simulink model "sv1_0"  (R2022b)
settings: Solver=VariableStepAuto  StartTime=0.0  StopTime=10.0  RelTol=1e-3
values from neighbouring files (symbols this model uses):
  m = rotation_matrix([0 0 1], theta)    [ectopic.m]    (also in ectopic_dirty_1.m; workspace.m)
undefined symbols (not defined in the file or in its folder): X, Y, Z
libraries: sm_lib x67, nesl_utility x1
(part 1 of 2)
settings Model: Creator=谢兴彪  LastModifiedBy=谢兴彪

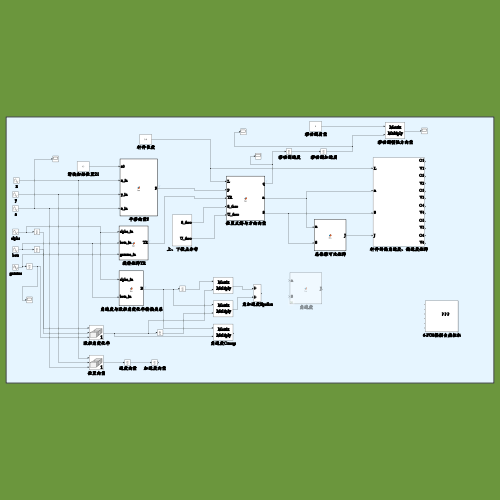
[thumbnail: Simulink's stored preview of the top-level diagram]
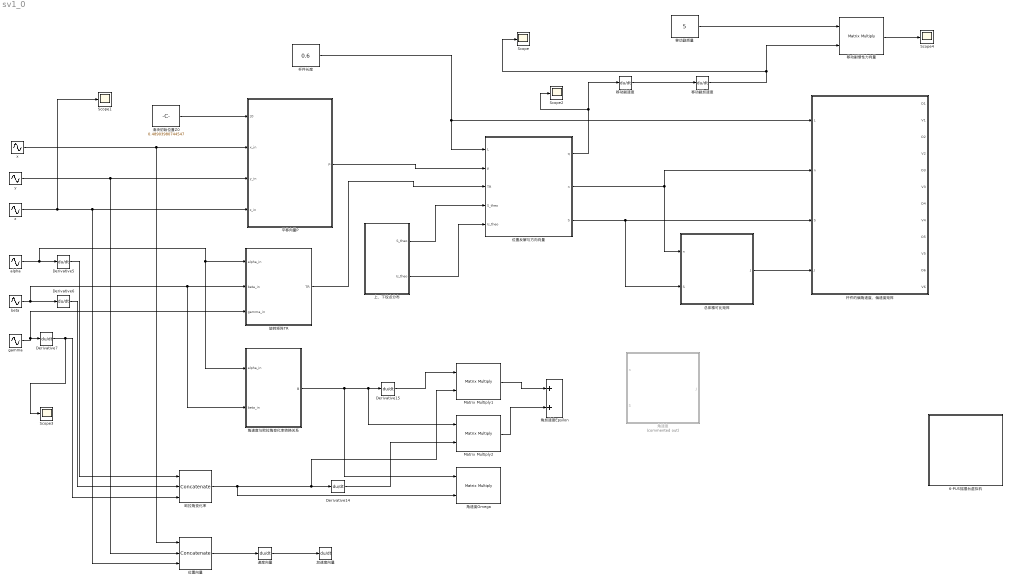
== system sv1_0 ==
  6-PUS摇摆台虚拟机 : Subsystem
      mask Display: image('C:\Users\谢兴彪\Desktop\微信图片_20230811154149.png'); % 使用工具条上的 "编辑图像" 进行更改。
  Derivative{5..7,14..15} (5 alike) : Derivative
  Matrix Multiply1 : Product  Inputs=**  Multiplication=Matrix(*)
  Matrix Multiply2 : Product  Inputs=**  Multiplication=Matrix(*)
  Scope{,1..4} (5 alike) : Scope
  alpha : Sin  Amplitude=0  Frequency=2*pi  SampleTime=0
  beta : Sin  Amplitude=0  Frequency=2*pi  SampleTime=0
  gamma : Sin  Amplitude=0.1  Frequency=2*pi  SampleTime=0.01
  x : Sin  Amplitude=0  Frequency=2*pi  SampleTime=0
  y : Sin  Amplitude=0  Frequency=2*pi  SampleTime=0
  z : Sin  Amplitude=0  Frequency=2  SampleTime=0
  上、下铰点分布 : Subsystem
  位置反解与方向向量 : MATLAB Function  TreatAsAtomicUnit=on
  位置向量 : Concatenate  NumInputs=3  Mode=Multidimensional array
  加速度向量 : Derivative
  平移向量P : MATLAB Function  TreatAsAtomicUnit=on
  总体雅可比矩阵 : MATLAB Function  TreatAsAtomicUnit=on
  旋转矩阵TR : MATLAB Function  TreatAsAtomicUnit=on
  杆件的偏角速度、偏速度矩阵 : Subsystem
  杆件长度 : Constant  Value=0.6
  欧拉角变化率 : Concatenate  NumInputs=3  Mode=Multidimensional array
  滑块初始位置Z0 : Constant  Value=0.48903980744547
  移动副加速度 : Derivative
  移动副惯性力向量 : Product  Inputs=**  Multiplication=Matrix(*)
  移动副质量 : Constant  Value=5
  移动副速度 : Derivative
  角加速度Epsilon : Sum
  角速度 : MATLAB Function  Commented=on  TreatAsAtomicUnit=on
  角速度Omega : Product  Inputs=**  Multiplication=Matrix(*)
  角速度与欧拉角变化率转换关系 : MATLAB Function  TreatAsAtomicUnit=on
  速度向量 : Derivative
  wires:
  滑块初始位置Z0/1 -> 平移向量P/1(z0)
  平移向量P/1(p) -> 位置反解与方向向量/2(p)
  旋转矩阵TR/1(TR) -> 位置反解与方向向量/3(TR)
  上、下铰点分布/1(S_theo) -> 位置反解与方向向量/4(S_theo)
  上、下铰点分布/2(U_theo) -> 位置反解与方向向量/5(U_theo)
  杆件长度/1 -> 位置反解与方向向量/1(L), 杆件的偏角速度、偏速度矩阵/1(L)
  位置反解与方向向量/1(q) -> 移动副速度/1, Scope2/1
  移动副速度/1 -> 移动副加速度/1
  z/1 -> Scope1/1, 位置向量/3, 平移向量P/4(z_in)
  y/1 -> 位置向量/2, 平移向量P/3(y_in)
  x/1 -> 平移向量P/2(x_in), 位置向量/1
  alpha/1 -> 角速度与欧拉角变化率转换关系/1(alpha_in), 旋转矩阵TR/1(alpha_in), Derivative5/1
  beta/1 -> 角速度与欧拉角变化率转换关系/2(beta_in), 旋转矩阵TR/2(beta_in), Derivative6/1
  gamma/1 -> 旋转矩阵TR/3(gamma_in), Derivative7/1
  Derivative5/1 -> 欧拉角变化率/1
  Derivative6/1 -> 欧拉角变化率/2
  Derivative7/1 -> Scope3/1, 欧拉角变化率/3
  欧拉角变化率/1 -> 角速度Omega/2, Matrix Multiply1/2, Derivative14/1
  Derivative14/1 -> Matrix Multiply2/2
  角速度与欧拉角变化率转换关系/1(B) -> Matrix Multiply2/1, Derivative15/1, 角速度Omega/1
  Derivative15/1 -> Matrix Multiply1/1
  Matrix Multiply1/1 -> 角加速度Epsilon/1
  Matrix Multiply2/1 -> 角加速度Epsilon/2
  位置向量/1 -> 速度向量/1
  速度向量/1 -> 加速度向量/1
  位置反解与方向向量/3(S) -> 总体雅可比矩阵/2(S), 杆件的偏角速度、偏速度矩阵/3(S)
  位置反解与方向向量/2(n) -> 杆件的偏角速度、偏速度矩阵/2(n), 总体雅可比矩阵/1(n)
  移动副质量/1 -> 移动副惯性力向量/1
  移动副加速度/1 -> 移动副惯性力向量/2, Scope/1
  总体雅可比矩阵/1(J) -> 杆件的偏角速度、偏速度矩阵/4(J)
  移动副惯性力向量/1 -> Scope4/1

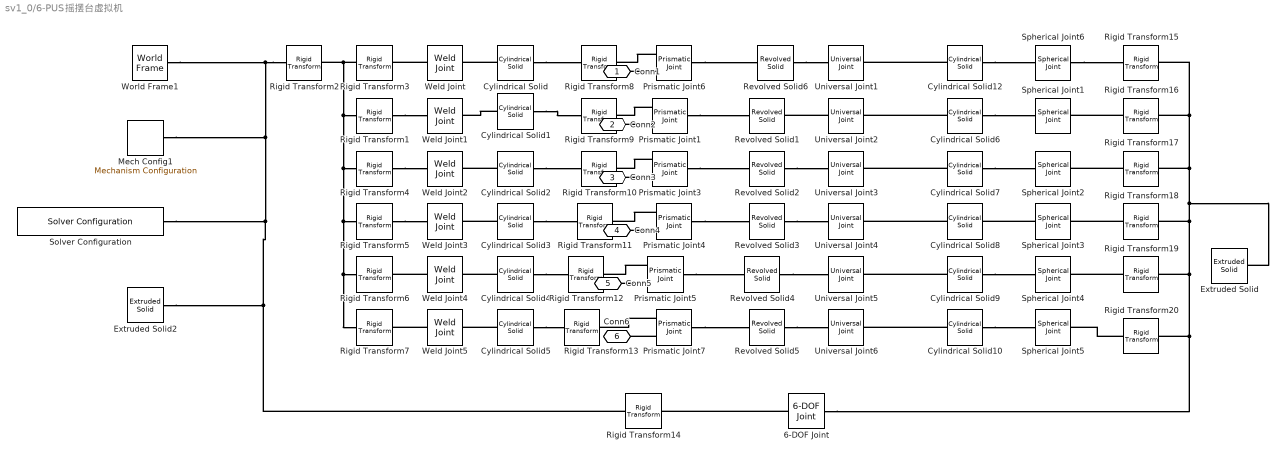
== system sv1_0/6-PUS摇摆台虚拟机 ==
  6-DOF Joint : sm_lib/Joints/6-DOF Joint  JointMode=Normal  SenseConstraintForce=off  SenseConstraintForceX=off  SenseConstraintForceY=off  SenseConstraintForceZ=off  SenseConstraintTorque=off  SenseConstraintTorqueX=off  SenseConstraintTorqueY=off  SenseConstraintTorqueZ=off  SenseTotalForce=off  SenseTotalForceX=off  SenseTotalForceY=off  SenseTotalForceZ=off  SenseTotalTorque=off  SenseTotalTorqueX=off  SenseTotalTorqueY=off  SenseTotalTorqueZ=off  CompositeWrenchDir=FollowerOnBase  CompositeWrenchFrame=BaseFrame  PxEquilibriumPosition=0  PxEquilibriumPositionUnits=m  PxSpringStiffness=0  PxSpringStiffnessUnits=N/m  PxDampingCoefficient=0  PxDampingCoefficientUnits=N/(m/s)  PxTorqueActuationMode=NoTorque  PxMotionActuationMode=ComputedMotion  PxSensePosition=off  PxSenseVelocity=off  PxSenseAcceleration=off  PxSenseTorqueForce=off  PxSenseLowerLimitTorqueForce=off  PxSenseUpperLimitTorqueForce=off  PxLowerLimitSpecify=off  PxLowerLimitBound=-1  PxLowerLimitBoundUnits=m  PxLowerLimitStiffness=1e6  PxLowerLimitStiffnessUnits=N/m  PxLowerLimitDamping=1e3  PxLowerLimitDampingUnits=N/(m/s)  PxLowerLimitTransitionRegionWidth=1e-4  PxLowerLimitTransitionRegionWidthUnits=m  PxUpperLimitSpecify=off  PxUpperLimitBound=1  PxUpperLimitBoundUnits=m  PxUpperLimitStiffness=1e6  PxUpperLimitStiffnessUnits=N/m  PxUpperLimitDamping=1e3  PxUpperLimitDampingUnits=N/(m/s)  PxUpperLimitTransitionRegionWidth=1e-4  PxUpperLimitTransitionRegionWidthUnits=m  PxPositionTargetSpecify=off  PxPositionTargetPriority=High  PxPositionTargetValue=0  PxPositionTargetValueUnits=m  PxVelocityTargetSpecify=off  PxVelocityTargetPriority=High  PxVelocityTargetValue=0  PxVelocityTargetValueUnits=m/s  PyEquilibriumPosition=0  PyEquilibriumPositionUnits=m  PySpringStiffness=0  PySpringStiffnessUnits=N/m  PyDampingCoefficient=0  PyDampingCoefficientUnits=N/(m/s)  PyTorqueActuationMode=NoTorque  PyMotionActuationMode=ComputedMotion  PySensePosition=off  PySenseVelocity=off  PySenseAcceleration=off  PySenseTorqueForce=off  PySenseLowerLimitTorqueForce=off  PySenseUpperLimitTorqueForce=off  PyLowerLimitSpecify=off  PyLowerLimitBound=-1  PyLowerLimitBoundUnits=m  PyLowerLimitStiffness=1e6  PyLowerLimitStiffnessUnits=N/m  PyLowerLimitDamping=1e3  PyLowerLimitDampingUnits=N/(m/s)  PyLowerLimitTransitionRegionWidth=1e-4  PyLowerLimitTransitionRegionWidthUnits=m  PyUpperLimitSpecify=off  PyUpperLimitBound=1  PyUpperLimitBoundUnits=m  PyUpperLimitStiffness=1e6  PyUpperLimitStiffnessUnits=N/m  PyUpperLimitDamping=1e3  PyUpperLimitDampingUnits=N/(m/s)  PyUpperLimitTransitionRegionWidth=1e-4  PyUpperLimitTransitionRegionWidthUnits=m  PyPositionTargetSpecify=off  PyPositionTargetPriority=High  PyPositionTargetValue=0  PyPositionTargetValueUnits=m  PyVelocityTargetSpecify=off  PyVelocityTargetPriority=High  PyVelocityTargetValue=0  PyVelocityTargetValueUnits=m/s  PzEquilibriumPosition=0  PzEquilibriumPositionUnits=m  PzSpringStiffness=0  PzSpringStiffnessUnits=N/m  PzDampingCoefficient=0  PzDampingCoefficientUnits=N/(m/s)  PzTorqueActuationMode=NoTorque  PzMotionActuationMode=ComputedMotion  PzSensePosition=off  PzSenseVelocity=off  PzSenseAcceleration=off  PzSenseTorqueForce=off  PzSenseLowerLimitTorqueForce=off  PzSenseUpperLimitTorqueForce=off  PzLowerLimitSpecify=off  PzLowerLimitBound=-1  PzLowerLimitBoundUnits=m  PzLowerLimitStiffness=1e6  PzLowerLimitStiffnessUnits=N/m  PzLowerLimitDamping=1e3  PzLowerLimitDampingUnits=N/(m/s)  PzLowerLimitTransitionRegionWidth=1e-4  PzLowerLimitTransitionRegionWidthUnits=m  PzUpperLimitSpecify=off  PzUpperLimitBound=1  PzUpperLimitBoundUnits=m  PzUpperLimitStiffness=1e6  PzUpperLimitStiffnessUnits=N/m  PzUpperLimitDamping=1e3  PzUpperLimitDampingUnits=N/(m/s)  PzUpperLimitTransitionRegionWidth=1e-4  PzUpperLimitTransitionRegionWidthUnits=m  PzPositionTargetSpecify=off  PzPositionTargetPriority=High  PzPositionTargetValue=0  PzPositionTargetValueUnits=m  PzVelocityTargetSpecify=off  PzVelocityTargetPriority=High  PzVelocityTargetValue=0  PzVelocityTargetValueUnits=m/s  SphEqPosRotationMethod=None  SphEqPosRotationAngleUnits=deg  SphEqPosRotationStandardAxis=+Z  SphEqPosRotationAngle=0.0  SphEqPosRotationArbitraryAxis=[0 0 1]  SphEqPosFollAlignAxisA=+X  SphEqPosBaseAlignAxisA=+Y  SphEqPosFollAlignAxisB=+Y  SphEqPosBaseAlignAxisB=+Z  SphEqPosRotationSequenceAxes=FollowerAxes  SphEqPosRotationSequence=XYX  SphEqPosRotationSequenceAngles=[0 0 0]  SphEqPosRotationSequenceAnglesUnits=deg  SphEqPosRotationMatrix=[1 0 0; 0 1 0; 0 0 1]  SphEqPosQuaternion=[1 0 0 0]  SphSpringStiffness=0  SphSpringStiffnessUnits=N*m/deg  SphDampingCoefficient=0  SphDampingCoefficientUnits=N*m/(deg/s)  SphActuateTorqueX=off  SphActuateTorqueY=off  SphActuateTorqueZ=off  SphActuateTorque=off  SphTorqueActuationMode=NoTorque  SphMotionActuationMode=ComputedMotion  SphActuationFrame=BaseFrame  SphSensePosition=off  SphSenseVelocityX=off  SphSenseVelocityY=off  SphSenseVelocityZ=off  SphSenseVelocity=off  SphSenseAccelerationX=off  SphSenseAccelerationY=off  SphSenseAccelerationZ=off  SphSenseAcceleration=off  SphSenseTorqueX=off  SphSenseTorqueY=off  SphSenseTorqueZ=off  SphSenseTorqueForce=off  SphSenseLowerLimitTorqueMag=off  SphSenseUpperLimitTorqueMag=off  SphSensingFrame=BaseFrame  SphLowerLimitSpecify=off  SphLowerLimitBound=15  SphLowerLimitBoundUnits=deg  SphLowerLimitStiffness=1e4  SphLowerLimitStiffnessUnits=N*m/deg  SphLowerLimitDamping=10  SphLowerLimitDampingUnits=N*m/(deg/s)  SphLowerLimitTransitionRegionWidth=0.1  SphLowerLimitTransitionRegionWidthUnits=deg  SphUpperLimitSpecify=off  SphUpperLimitBound=45  SphUpperLimitBoundUnits=deg  SphUpperLimitStiffness=1e4  SphUpperLimitStiffnessUnits=N*m/deg  SphUpperLimitDamping=10  SphUpperLimitDampingUnits=N*m/(deg/s)  SphUpperLimitTransitionRegionWidth=0.1  SphUpperLimitTransitionRegionWidthUnits=deg  SphPositionTargetRotationMethod=None  SphPositionTargetRotationAngleUnits=deg  SphPositionTargetRotationStandardAxis=+Z  SphPositionTargetRotationAngle=0.0  SphPositionTargetRotationArbitraryAxis=[0 0 1]  SphPositionTargetFollAlignAxisA=+X  SphPositionTargetBaseAlignAxisA=+Y  SphPositionTargetFollAlignAxisB=+Y  SphPositionTargetBaseAlignAxisB=+Z  SphPositionTargetRotationSequenceAxes=FollowerAxes  SphPositionTargetRotationSequence=XYX  SphPositionTargetRotationSequenceAngles=[0 0 0]  SphPositionTargetRotationSequenceAnglesUnits=deg  SphPositionTargetRotationMatrix=[1 0 0; 0 1 0; 0 0 1]  SphPositionTargetQuaternion=[1 0 0 0]  SphPositionTargetSpecify=off  SphPositionTargetPriority=High  SphVelocityTargetValue=[0 0 0]  SphVelocityTargetValueUnits=deg/s  SphVelocityTargetSpecify=off  SphVelocityTargetPriority=High  SphVelocityTargetInFollowerFrame=on
  Cylindrical Solid{,1..5} (6 alike) : sm_lib/Body Elements/Cylindrical Solid  GraphicAmbientColor=[0.15 0.15 0.15 1.0]  BasedOnType=Density  CenterOfMass=[0 0 0]  CenterOfMassUnits=m  GraphicDiffuseColor=[1 0.4 0.0]  CylinderLength=536.5  CylinderLengthUnits=mm  CylinderRadius=7.5  CylinderRadiusUnits=mm  Density=1000  DensityUnits=kg/m^3  DoExposeReferenceFrame=off  GraphicEmissiveColor=[0.0 0.0 0.0 1.0]  ExportEntireGeometry=off  SerializedFrames=<Frames><Frame><Id>Frame1</Id><Value><Name>F1</Name><Origin><Source>GeometricFeature</Source><FeatureName>bottom curve</FeatureName></Origin><PrimaryAxis><DefinedDirection>+Z</DefinedDirection><Source>ReferenceFrame</Source><SourceDirection>+Z</SourceDirection><FeatureName></FeatureName></PrimaryAxis><SecondaryAxis><DefinedDirection>+X</DefinedDirection><Source>ReferenceFrame</Source><SourceDirection>+X</SourceDirection><FeatureName></FeatureName></SecondaryAxis></Value></Frame><Frame><Id>Frame2</Id><Value><Name>F2</Name><Origin><Source>GeometricFeature</Source><FeatureName>top surface</FeatureName></Origin><PrimaryAxis><DefinedDirection>+Z</DefinedDirection><Source>ReferenceFrame</Source><SourceDirection>+Z</SourceDirection><FeatureName></FeatureName></PrimaryAxis><SecondaryAxis><DefinedDirection>+X</DefinedDirection><Source>ReferenceFrame</Source><SourceDirection>+X</SourceDirection><FeatureName></FeatureName></SecondaryAxis></Value></Frame></Frames>  MarkerShape=Sphere  MarkerSize=10  GraphicType=FromGeometry  InertiaType=CalculateFromGeometry  Mass=1  MassUnits=kg  MomentsOfInertia=[1 1 1]  MomentsOfInertiaUnits=kg*m^2  GraphicOpacity=1.0  ProductsOfInertia=[0 0 0]  ProductsOfInertiaUnits=kg*m^2  GraphicShininess=75  GraphicSpecularColor=[0.5 0.5 0.5 1.0]  GraphicVisPropType=SimpleVisualProperties
  Cylindrical Solid{6..10,12} (6 alike) : sm_lib/Body Elements/Cylindrical Solid  GraphicAmbientColor=[0.15 0.15 0.15 1.0]  BasedOnType=Density  CenterOfMass=[0 0 0]  CenterOfMassUnits=m  GraphicDiffuseColor=[1.0 0.2 0.0]  CylinderLength=600  CylinderLengthUnits=mm  CylinderRadius=20  CylinderRadiusUnits=mm  Density=1000  DensityUnits=kg/m^3  DoExposeReferenceFrame=off  GraphicEmissiveColor=[0.0 0.0 0.0 1.0]  ExportEntireGeometry=off  SerializedFrames=<Frames><Frame><Id>Frame1</Id><Value><Name>F1</Name><Origin><Source>GeometricFeature</Source><FeatureName>bottom curve</FeatureName></Origin><PrimaryAxis><DefinedDirection>+Z</DefinedDirection><Source>ReferenceFrame</Source><SourceDirection>+Z</SourceDirection><FeatureName></FeatureName></PrimaryAxis><SecondaryAxis><DefinedDirection>+X</DefinedDirection><Source>ReferenceFrame</Source><SourceDirection>+X</SourceDirection><FeatureName></FeatureName></SecondaryAxis></Value></Frame><Frame><Id>Frame2</Id><Value><Name>F2</Name><Origin><Source>GeometricFeature</Source><FeatureName>top surface</FeatureName></Origin><PrimaryAxis><DefinedDirection>+Z</DefinedDirection><Source>ReferenceFrame</Source><SourceDirection>+Z</SourceDirection><FeatureName></FeatureName></PrimaryAxis><SecondaryAxis><DefinedDirection>+X</DefinedDirection><Source>ReferenceFrame</Source><SourceDirection>+X</SourceDirection><FeatureName></FeatureName></SecondaryAxis></Value></Frame></Frames>  MarkerShape=Sphere  MarkerSize=10  GraphicType=FromGeometry  InertiaType=CalculateFromGeometry  Mass=1  MassUnits=kg  MomentsOfInertia=[1 1 1]  MomentsOfInertiaUnits=kg*m^2  GraphicOpacity=1.0  ProductsOfInertia=[0 0 0]  ProductsOfInertiaUnits=kg*m^2  GraphicShininess=75  GraphicSpecularColor=[0.5 0.5 0.5 1.0]  GraphicVisPropType=SimpleVisualProperties
  Extruded Solid : sm_lib/Body Elements/Extruded Solid  GraphicAmbientColor=[0.15 0.15 0.15 1.0]  BasedOnType=Density  CenterOfMass=[0 0 0]  CenterOfMassUnits=m  GraphicDiffuseColor=[0 0.1 1]  ExportConvexHullGeometry=off  ExtrusionCrossSection=|  ExtrusionCrossSectionUnits=m  Density=1000  DensityUnits=kg/m^3  DoExposeReferenceFrame=on  GraphicEmissiveColor=[0.0 0.0 0.0 0.3]  ExportEntireGeometry=off  ExtrusionLength=0.025  ExtrusionLengthUnits=m  ExtrusionType=General  SerializedFrames=<Frames/>  MarkerShape=Sphere  MarkerSize=10  GraphicType=FromGeometry  InertiaType=CalculateFromGeometry  Mass=1  MassUnits=kg  MomentsOfInertia=[1 1 1]  MomentsOfInertiaUnits=kg*m^2  PolygonNumSides=6  GraphicOpacity=1.0  PolygonOuterRadius=0.16  PolygonOuterRadiusUnits=m  ProductsOfInertia=[0 0 0]  ProductsOfInertiaUnits=kg*m^2  GraphicShininess=75  GraphicSpecularColor=[0.5 0.5 0.5 1.0]  GraphicVisPropType=AdvancedVisualProperties
      | [0.1373 0.1314; 
      | -0.1373 0.1314; 
      | -0.1824 0.0532; 
      | -0.0451 -0.1846;
      | 0.0451 -0.1846;
      | 0.1824 0.0532]
  Extruded Solid2 : sm_lib/Body Elements/Extruded Solid  GraphicAmbientColor=[0.15 0.15 0.15 1.0]  BasedOnType=Density  CenterOfMass=[0 0 0]  CenterOfMassUnits=m  GraphicDiffuseColor=[1 0.4 0]  ExportConvexHullGeometry=off  ExtrusionCrossSection=|  ExtrusionCrossSectionUnits=m  Density=1000  DensityUnits=kg/m^3  DoExposeReferenceFrame=on  GraphicEmissiveColor=[0.0 0.0 0.0 0.3]  ExportEntireGeometry=off  ExtrusionLength=0.2  ExtrusionLengthUnits=m  ExtrusionType=General  SerializedFrames=<Frames/>  MarkerShape=Sphere  MarkerSize=10  GraphicType=FromGeometry  InertiaType=CalculateFromGeometry  Mass=1  MassUnits=kg  MomentsOfInertia=[1 1 1]  MomentsOfInertiaUnits=kg*m^2  PolygonNumSides=6  GraphicOpacity=1.0  PolygonOuterRadius=0.16  PolygonOuterRadiusUnits=m  ProductsOfInertia=[0 0 0]  ProductsOfInertiaUnits=kg*m^2  GraphicShininess=75  GraphicSpecularColor=[0.5 0.5 0.5 1.0]  GraphicVisPropType=AdvancedVisualProperties
      | [0.1096 0.4878; 
      | -0.1096 0.4878; 
      | -0.4773 -0.1490; 
      | -0.3677 -0.3388;
      | 0.3677 -0.3388;
      | 0.4773 -0.1490]
  Mech Config1 : sm_lib/Utilities/Mechanism Configuration  UniformGravity=None  GravityVector=[0 0 -9.80665]  GravityUnits=m/s^2  LinearizationDelta=0.001  JointModeTransitionNonlinearIterations=2
  Prismatic Joint{1,3..7} (6 alike) : sm_lib/Joints/Prismatic Joint  JointMode=Normal  SenseConstraintForce=off  SenseConstraintForceX=off  SenseConstraintForceY=off  SenseConstraintForceZ=off  SenseConstraintTorque=off  SenseConstraintTorqueX=off  SenseConstraintTorqueY=off  SenseConstraintTorqueZ=off  SenseTotalForce=off  SenseTotalForceX=off  SenseTotalForceY=off  SenseTotalForceZ=off  SenseTotalTorque=off  SenseTotalTorqueX=off  SenseTotalTorqueY=off  SenseTotalTorqueZ=off  CompositeWrenchDir=FollowerOnBase  CompositeWrenchFrame=BaseFrame  EquilibriumPosition=0  EquilibriumPositionUnits=m  SpringStiffness=10  SpringStiffnessUnits=N/m  DampingCoefficient=1  DampingCoefficientUnits=N/(m/s)  TorqueActuationMode=ComputedTorque  MotionActuationMode=InputMotion  SensePosition=off  SenseVelocity=off  SenseAcceleration=off  SenseTorqueForce=off  SenseLowerLimitTorqueForce=off  SenseUpperLimitTorqueForce=off  LowerLimitSpecify=off  LowerLimitBound=-1  LowerLimitBoundUnits=m  LowerLimitStiffness=1e6  LowerLimitStiffnessUnits=N/m  LowerLimitDamping=1e3  LowerLimitDampingUnits=N/(m/s)  LowerLimitTransitionRegionWidth=1e-4  LowerLimitTransitionRegionWidthUnits=m  UpperLimitSpecify=off  UpperLimitBound=1  UpperLimitBoundUnits=m  UpperLimitStiffness=1e6  UpperLimitStiffnessUnits=N/m  UpperLimitDamping=1e3  UpperLimitDampingUnits=N/(m/s)  UpperLimitTransitionRegionWidth=1e-4  UpperLimitTransitionRegionWidthUnits=m  PositionTargetSpecify=off  PositionTargetPriority=High  PositionTargetValue=0  PositionTargetValueUnits=m  VelocityTargetSpecify=off  VelocityTargetPriority=High  VelocityTargetValue=0  VelocityTargetValueUnits=m/s
  Revolved Solid{1..5} (5 alike) : sm_lib/Body Elements/Revolved Solid  GraphicAmbientColor=[0.15 0.15 0.15 1.0]  BasedOnType=Density  CenterOfMass=[0 0 0]  CenterOfMassUnits=m  GraphicDiffuseColor=[1.0 0.4 0]  ExportConvexHullGeometry=off  Density=1000  DensityUnits=kg/m^3  DoExposeReferenceFrame=on  GraphicEmissiveColor=[0.0 0.0 0.0 1.0]  ExportEntireGeometry=off  SerializedFrames=<Frames><Frame><Id>Frame1</Id><Value><Name>F1</Name><Origin><Source>GeometricFeature</Source><FeatureName>side surface 3</FeatureName></Origin><PrimaryAxis><DefinedDirection>+Z</DefinedDirection><Source>ReferenceFrame</Source><SourceDirection>+Z</SourceDirection><FeatureName></FeatureName></PrimaryAxis><SecondaryAxis><DefinedDirection>+X</DefinedDirection><Source>ReferenceFrame</Source><SourceDirection>+X</SourceDirection><FeatureName></FeatureName></SecondaryAxis></Value></Frame></Frames>  MarkerShape=Sphere  MarkerSize=10  GraphicType=FromGeometry  InertiaType=CalculateFromGeometry  Mass=1  MassUnits=kg  MomentsOfInertia=[1 1 1]  MomentsOfInertiaUnits=kg*m^2  GraphicOpacity=1.0  ProductsOfInertia=[0 0 0]  ProductsOfInertiaUnits=kg*m^2  RevolutionCrossSection=[3.75 10; 3.75 -10; 10 -10; 10 10]  RevolutionCrossSectionUnits=mm  RevolutionAngle=180  RevolutionAngleUnits=deg  RevolutionExtent=Full  GraphicShininess=75  GraphicSpecularColor=[0.5 0.5 0.5 1.0]  GraphicVisPropType=SimpleVisualProperties
  Revolved Solid6 : sm_lib/Body Elements/Revolved Solid  GraphicAmbientColor=[0.15 0.15 0.15 1.0]  BasedOnType=Density  CenterOfMass=[0 0 0]  CenterOfMassUnits=m  GraphicDiffuseColor=[0.0 0.6 0.0]  ExportConvexHullGeometry=off  Density=1000  DensityUnits=kg/m^3  DoExposeReferenceFrame=on  GraphicEmissiveColor=[0.0 0.0 0.0 1.0]  ExportEntireGeometry=off  SerializedFrames=<Frames><Frame><Id>Frame1</Id><Value><Name>F1</Name><Origin><Source>GeometricFeature</Source><FeatureName>side surface 3</FeatureName></Origin><PrimaryAxis><DefinedDirection>+Z</DefinedDirection><Source>ReferenceFrame</Source><SourceDirection>+Z</SourceDirection><FeatureName></FeatureName></PrimaryAxis><SecondaryAxis><DefinedDirection>+X</DefinedDirection><Source>ReferenceFrame</Source><SourceDirection>+X</SourceDirection><FeatureName></FeatureName></SecondaryAxis></Value></Frame></Frames>  MarkerShape=Sphere  MarkerSize=10  GraphicType=FromGeometry  InertiaType=CalculateFromGeometry  Mass=1  MassUnits=kg  MomentsOfInertia=[1 1 1]  MomentsOfInertiaUnits=kg*m^2  GraphicOpacity=1.0  ProductsOfInertia=[0 0 0]  ProductsOfInertiaUnits=kg*m^2  RevolutionCrossSection=[3.75 10; 3.75 -10; 10 -10; 10 10]  RevolutionCrossSectionUnits=mm  RevolutionAngle=180  RevolutionAngleUnits=deg  RevolutionExtent=Full  GraphicShininess=75  GraphicSpecularColor=[0.5 0.5 0.5 1.0]  GraphicVisPropType=SimpleVisualProperties
  Rigid Transform1 : sm_lib/Frames and Transforms/Rigid Transform  TranslationMethod=Cartesian  TranslationStandardOffset=0.1  TranslationLengthUnit=m  TranslationStandardAxis=+Z  TranslationCartesianOffset=[-0.086 0.457 0]  TranslationROffset=0  TranslationROffsetUnits=m  TranslationZOffset=0  TranslationZOffsetUnits=m  TranslationThetaOffset=0  TranslationThetaOffsetUnits=deg  RotationMethod=None  RotationAngleUnits=deg  RotationStandardAxis=+Z  RotationAngle=0.0  RotationArbitraryAxis=[0 0 1]  FollAlignAxisA=+X  BaseAlignAxisA=+Y  FollAlignAxisB=+Y  BaseAlignAxisB=+Z  RotationSequenceAxes=FollowerAxes  RotationSequence=XYX  RotationSequenceAngles=[0 0 0]  RotationSequenceAnglesUnits=deg  RotationMatrix=[1 0 0; 0 1 0; 0 0 1]  Quaternion=[1 0 0 0]
  Rigid Transform{8..13} (6 alike) : sm_lib/Frames and Transforms/Rigid Transform  TranslationMethod=StandardAxis  TranslationStandardOffset=0.3065  TranslationLengthUnit=m  TranslationStandardAxis=-Z  TranslationCartesianOffset=[0 0 0]  TranslationROffset=0  TranslationROffsetUnits=m  TranslationZOffset=0  TranslationZOffsetUnits=m  TranslationThetaOffset=0  TranslationThetaOffsetUnits=deg  RotationMethod=None  RotationAngleUnits=deg  RotationStandardAxis=+Z  RotationAngle=0.0  RotationArbitraryAxis=[0 0 1]  FollAlignAxisA=+X  BaseAlignAxisA=+Y  FollAlignAxisB=+Y  BaseAlignAxisB=+Z  RotationSequenceAxes=FollowerAxes  RotationSequence=XYX  RotationSequenceAngles=[0 0 0]  RotationSequenceAnglesUnits=deg  RotationMatrix=[1 0 0; 0 1 0; 0 0 1]  Quaternion=[1 0 0 0]
  Rigid Transform14 : sm_lib/Frames and Transforms/Rigid Transform  TranslationMethod=StandardAxis  TranslationStandardOffset=0.609  TranslationLengthUnit=m  TranslationStandardAxis=+Z  TranslationCartesianOffset=[0.4388 -0.1540 0]  TranslationROffset=0  TranslationROffsetUnits=m  TranslationZOffset=0  TranslationZOffsetUnits=m  TranslationThetaOffset=0  TranslationThetaOffsetUnits=deg  RotationMethod=None  RotationAngleUnits=deg  RotationStandardAxis=+Z  RotationAngle=0.0  RotationArbitraryAxis=[0 0 1]  FollAlignAxisA=+X  BaseAlignAxisA=+Y  FollAlignAxisB=+Y  BaseAlignAxisB=+Z  RotationSequenceAxes=FollowerAxes  RotationSequence=XYX  RotationSequenceAngles=[0 0 0]  RotationSequenceAnglesUnits=deg  RotationMatrix=[1 0 0; 0 1 0; 0 0 1]  Quaternion=[1 0 0 0]
  Rigid Transform15 : sm_lib/Frames and Transforms/Rigid Transform  TranslationMethod=Cartesian  TranslationStandardOffset=0.1  TranslationLengthUnit=m  TranslationStandardAxis=+Z  TranslationCartesianOffset=[0.1156 0.1106 0]  TranslationROffset=0  TranslationROffsetUnits=m  TranslationZOffset=0  TranslationZOffsetUnits=m  TranslationThetaOffset=0  TranslationThetaOffsetUnits=deg  RotationMethod=AlignedAxes  RotationAngleUnits=deg  RotationStandardAxis=+Z  RotationAngle=0.0  RotationArbitraryAxis=[0 0 1]  FollAlignAxisA=+X  BaseAlignAxisA=+Y  FollAlignAxisB=+Y  BaseAlignAxisB=+Z  RotationSequenceAxes=FollowerAxes  RotationSequence=XYX  RotationSequenceAngles=[0 0 0]  RotationSequenceAnglesUnits=deg  RotationMatrix=[1 0 0; 0 1 0; 0 0 1]  Quaternion=[1 0 0 0]
  Rigid Transform16 : sm_lib/Frames and Transforms/Rigid Transform  TranslationMethod=Cartesian  TranslationStandardOffset=0.1  TranslationLengthUnit=m  TranslationStandardAxis=+Z  TranslationCartesianOffset=[-0.1156 0.1106 0]  TranslationROffset=0  TranslationROffsetUnits=m  TranslationZOffset=0  TranslationZOffsetUnits=m  TranslationThetaOffset=0  TranslationThetaOffsetUnits=deg  RotationMethod=AlignedAxes  RotationAngleUnits=deg  RotationStandardAxis=+Z  RotationAngle=0.0  RotationArbitraryAxis=[0 0 1]  FollAlignAxisA=+X  BaseAlignAxisA=+Y  FollAlignAxisB=+Y  BaseAlignAxisB=+Z  RotationSequenceAxes=FollowerAxes  RotationSequence=XYX  RotationSequenceAngles=[0 0 0]  RotationSequenceAnglesUnits=deg  RotationMatrix=[1 0 0; 0 1 0; 0 0 1]  Quaternion=[1 0 0 0]
  Rigid Transform17 : sm_lib/Frames and Transforms/Rigid Transform  TranslationMethod=Cartesian  TranslationStandardOffset=0.1  TranslationLengthUnit=m  TranslationStandardAxis=+Z  TranslationCartesianOffset=[-0.1536 0.0448 0]  TranslationROffset=0  TranslationROffsetUnits=m  TranslationZOffset=0  TranslationZOffsetUnits=m  TranslationThetaOffset=0  TranslationThetaOffsetUnits=deg  RotationMethod=AlignedAxes  RotationAngleUnits=deg  RotationStandardAxis=+Z  RotationAngle=0.0  RotationArbitraryAxis=[0 0 1]  FollAlignAxisA=+X  BaseAlignAxisA=+Y  FollAlignAxisB=+Y  BaseAlignAxisB=+Z  RotationSequenceAxes=FollowerAxes  RotationSequence=XYX  RotationSequenceAngles=[0 0 0]  RotationSequenceAnglesUnits=deg  RotationMatrix=[1 0 0; 0 1 0; 0 0 1]  Quaternion=[1 0 0 0]
  Rigid Transform18 : sm_lib/Frames and Transforms/Rigid Transform  TranslationMethod=Cartesian  TranslationStandardOffset=0.1  TranslationLengthUnit=m  TranslationStandardAxis=+Z  TranslationCartesianOffset="[-0.038  -0.1554 0]"  TranslationROffset=0  TranslationROffsetUnits=m  TranslationZOffset=0  TranslationZOffsetUnits=m  TranslationThetaOffset=0  TranslationThetaOffsetUnits=deg  RotationMethod=AlignedAxes  RotationAngleUnits=deg  RotationStandardAxis=+Z  RotationAngle=0.0  RotationArbitraryAxis=[0 0 1]  FollAlignAxisA=+X  BaseAlignAxisA=+Y  FollAlignAxisB=+Y  BaseAlignAxisB=+Z  RotationSequenceAxes=FollowerAxes  RotationSequence=XYX  RotationSequenceAngles=[0 0 0]  RotationSequenceAnglesUnits=deg  RotationMatrix=[1 0 0; 0 1 0; 0 0 1]  Quaternion=[1 0 0 0]
  Rigid Transform19 : sm_lib/Frames and Transforms/Rigid Transform  TranslationMethod=Cartesian  TranslationStandardOffset=0.1  TranslationLengthUnit=m  TranslationStandardAxis=+Z  TranslationCartesianOffset=[0.038 -0.1554 0]  TranslationROffset=0  TranslationROffsetUnits=m  TranslationZOffset=0  TranslationZOffsetUnits=m  TranslationThetaOffset=0  TranslationThetaOffsetUnits=deg  RotationMethod=AlignedAxes  RotationAngleUnits=deg  RotationStandardAxis=+Z  RotationAngle=0.0  RotationArbitraryAxis=[0 0 1]  FollAlignAxisA=+X  BaseAlignAxisA=+Y  FollAlignAxisB=+Y  BaseAlignAxisB=+Z  RotationSequenceAxes=FollowerAxes  RotationSequence=XYX  RotationSequenceAngles=[0 0 0]  RotationSequenceAnglesUnits=deg  RotationMatrix=[1 0 0; 0 1 0; 0 0 1]  Quaternion=[1 0 0 0]
  Rigid Transform2 : sm_lib/Frames and Transforms/Rigid Transform  TranslationMethod=StandardAxis  TranslationStandardOffset=0.1  TranslationLengthUnit=m  TranslationStandardAxis=+Z  TranslationCartesianOffset=[0 0 0]  TranslationROffset=0  TranslationROffsetUnits=m  TranslationZOffset=0  TranslationZOffsetUnits=m  TranslationThetaOffset=0  TranslationThetaOffsetUnits=deg  RotationMethod=None  RotationAngleUnits=deg  RotationStandardAxis=+Z  RotationAngle=0.0  RotationArbitraryAxis=[0 0 1]  FollAlignAxisA=+X  BaseAlignAxisA=+Y  FollAlignAxisB=+Y  BaseAlignAxisB=+Z  RotationSequenceAxes=FollowerAxes  RotationSequence=XYX  RotationSequenceAngles=[0 0 0]  RotationSequenceAnglesUnits=deg  RotationMatrix=[1 0 0; 0 1 0; 0 0 1]  Quaternion=[1 0 0 0]
  Rigid Transform20 : sm_lib/Frames and Transforms/Rigid Transform  TranslationMethod=Cartesian  TranslationStandardOffset=0.1  TranslationLengthUnit=m  TranslationStandardAxis=+Z  TranslationCartesianOffset=[0.15336 0.0448 0]  TranslationROffset=0  TranslationROffsetUnits=m  TranslationZOffset=0  TranslationZOffsetUnits=m  TranslationThetaOffset=0  TranslationThetaOffsetUnits=deg  RotationMethod=AlignedAxes  RotationAngleUnits=deg  RotationStandardAxis=+Z  RotationAngle=0.0  RotationArbitraryAxis=[0 0 1]  FollAlignAxisA=+X  BaseAlignAxisA=+Y  FollAlignAxisB=+Y  BaseAlignAxisB=+Z  RotationSequenceAxes=FollowerAxes  RotationSequence=XYX  RotationSequenceAngles=[0 0 0]  RotationSequenceAnglesUnits=deg  RotationMatrix=[1 0 0; 0 1 0; 0 0 1]  Quaternion=[1 0 0 0]
  Rigid Transform3 : sm_lib/Frames and Transforms/Rigid Transform  TranslationMethod=Cartesian  TranslationStandardOffset=0.1  TranslationLengthUnit=m  TranslationStandardAxis=+Z  TranslationCartesianOffset=[0.086 0.457 0]  TranslationROffset=0  TranslationROffsetUnits=m  TranslationZOffset=0  TranslationZOffsetUnits=m  TranslationThetaOffset=0  TranslationThetaOffsetUnits=deg  RotationMethod=None  RotationAngleUnits=deg  RotationStandardAxis=+Z  RotationAngle=0.0  RotationArbitraryAxis=[0 0 1]  FollAlignAxisA=+X  BaseAlignAxisA=+Y  FollAlignAxisB=+Y  BaseAlignAxisB=+Z  RotationSequenceAxes=FollowerAxes  RotationSequence=XYX  RotationSequenceAngles=[0 0 0]  RotationSequenceAnglesUnits=deg  RotationMatrix=[1 0 0; 0 1 0; 0 0 1]  Quaternion=[1 0 0 0]
  Rigid Transform4 : sm_lib/Frames and Transforms/Rigid Transform  TranslationMethod=Cartesian  TranslationStandardOffset=0.1  TranslationLengthUnit=m  TranslationStandardAxis=+Z  TranslationCartesianOffset=[-0.4388 -0.1540 0]  TranslationROffset=0  TranslationROffsetUnits=m  TranslationZOffset=0  TranslationZOffsetUnits=m  TranslationThetaOffset=0  TranslationThetaOffsetUnits=deg  RotationMethod=None  RotationAngleUnits=deg  RotationStandardAxis=+Z  RotationAngle=0.0  RotationArbitraryAxis=[0 0 1]  FollAlignAxisA=+X  BaseAlignAxisA=+Y  FollAlignAxisB=+Y  BaseAlignAxisB=+Z  RotationSequenceAxes=FollowerAxes  RotationSequence=XYX  RotationSequenceAngles=[0 0 0]  RotationSequenceAnglesUnits=deg  RotationMatrix=[1 0 0; 0 1 0; 0 0 1]  Quaternion=[1 0 0 0]
  Rigid Transform5 : sm_lib/Frames and Transforms/Rigid Transform  TranslationMethod=Cartesian  TranslationStandardOffset=0.1  TranslationLengthUnit=m  TranslationStandardAxis=+Z  TranslationCartesianOffset=[-0.3528 -0.3030 0]  TranslationROffset=0  TranslationROffsetUnits=m  TranslationZOffset=0  TranslationZOffsetUnits=m  TranslationThetaOffset=0  TranslationThetaOffsetUnits=deg  RotationMethod=None  RotationAngleUnits=deg  RotationStandardAxis=+Z  RotationAngle=0.0  RotationArbitraryAxis=[0 0 1]  FollAlignAxisA=+X  BaseAlignAxisA=+Y  FollAlignAxisB=+Y  BaseAlignAxisB=+Z  RotationSequenceAxes=FollowerAxes  RotationSequence=XYX  RotationSequenceAngles=[0 0 0]  RotationSequenceAnglesUnits=deg  RotationMatrix=[1 0 0; 0 1 0; 0 0 1]  Quaternion=[1 0 0 0]
  Rigid Transform6 : sm_lib/Frames and Transforms/Rigid Transform  TranslationMethod=Cartesian  TranslationStandardOffset=0.1  TranslationLengthUnit=m  TranslationStandardAxis=+Z  TranslationCartesianOffset=[0.3528 -0.3030 0]  TranslationROffset=0  TranslationROffsetUnits=m  TranslationZOffset=0  TranslationZOffsetUnits=m  TranslationThetaOffset=0  TranslationThetaOffsetUnits=deg  RotationMethod=None  RotationAngleUnits=deg  RotationStandardAxis=+Z  RotationAngle=0.0  RotationArbitraryAxis=[0 0 1]  FollAlignAxisA=+X  BaseAlignAxisA=+Y  FollAlignAxisB=+Y  BaseAlignAxisB=+Z  RotationSequenceAxes=FollowerAxes  RotationSequence=XYX  RotationSequenceAngles=[0 0 0]  RotationSequenceAnglesUnits=deg  RotationMatrix=[1 0 0; 0 1 0; 0 0 1]  Quaternion=[1 0 0 0]
  Rigid Transform7 : sm_lib/Frames and Transforms/Rigid Transform  TranslationMethod=Cartesian  TranslationStandardOffset=0.1  TranslationLengthUnit=m  TranslationStandardAxis=+Z  TranslationCartesianOffset=[0.4388 -0.1540 0]  TranslationROffset=0  TranslationROffsetUnits=m  TranslationZOffset=0  TranslationZOffsetUnits=m  TranslationThetaOffset=0  TranslationThetaOffsetUnits=deg  RotationMethod=None  RotationAngleUnits=deg  RotationStandardAxis=+Z  RotationAngle=0.0  RotationArbitraryAxis=[0 0 1]  FollAlignAxisA=+X  BaseAlignAxisA=+Y  FollAlignAxisB=+Y  BaseAlignAxisB=+Z  RotationSequenceAxes=FollowerAxes  RotationSequence=XYX  RotationSequenceAngles=[0 0 0]  RotationSequenceAnglesUnits=deg  RotationMatrix=[1 0 0; 0 1 0; 0 0 1]  Quaternion=[1 0 0 0]
  Solver Configuration : nesl_utility/Solver Configuration  PhysicalDomain=network_engine_domain  SubClassName=solver  LeftPortType=input  RightPortType=generic  Tones=[]  Harmonics=[]  SimulateNoise=off  Profile=off  UseLocalSampling=off  EnableSwitchedLinearOptims=on  FrequencyDomain=off  UseCCode=off  RelTol=0.001  AbsTol=0.001  MinStep=1e-09  ToWorkspace=off  RevertToSquareIcSolve=off  NumHomotopyIterations=100  PhasorMode=off  PhasorModeNumHarmonics=1  ConsistencySolver=NEWTON_XTOL_AFTER_FTOL  IndexReductionMethod=DerivativeReplacement  DoDC=off  ResidualTolerance=1e-09  ConsistencyTolSource=GLOBAL  ConsistencyAbsTol=0.001  ConsistencyRelTol=0.001  ConsistencyTolFactor=0.001  UseLocalSolver=off  LocalSolverChoice=NE_BACKWARD_EULER_ADVANCER  ResolveIndetEquations=on  FunctionEvalNumThread=1  LocalSolverSampleTime=0.001  DoFixedCost=off  MaxNonlinIter=3  MaxModeIter=2  ComputeImpulses=off  ImpulseIterations=2  LinearAlgebra=auto  LinearAlgebraNumThread=0  EquationFormulation=NE_TIME_EF  DelaysMemoryBudget=1024  AutomaticFiltering=on  FilteringTimeConstant=0.001  PartitionStorageMethod=AS_NEEDED  PartitionMemoryBudget=1024  PartitionMethod=ROBUST
  Spherical Joint{1..6} (6 alike) : sm_lib/Joints/Spherical Joint  JointMode=Normal  SenseConstraintForce=off  SenseConstraintForceX=off  SenseConstraintForceY=off  SenseConstraintForceZ=off  SenseConstraintTorque=off  SenseConstraintTorqueX=off  SenseConstraintTorqueY=off  SenseConstraintTorqueZ=off  SenseTotalForce=off  SenseTotalForceX=off  SenseTotalForceY=off  SenseTotalForceZ=off  SenseTotalTorque=off  SenseTotalTorqueX=off  SenseTotalTorqueY=off  SenseTotalTorqueZ=off  CompositeWrenchDir=FollowerOnBase  CompositeWrenchFrame=BaseFrame  EqPosRotationMethod=None  EqPosRotationAngleUnits=deg  EqPosRotationStandardAxis=+Z  EqPosRotationAngle=0.0  EqPosRotationArbitraryAxis=[0 0 1]  EqPosFollAlignAxisA=+X  EqPosBaseAlignAxisA=+Y  EqPosFollAlignAxisB=+Y  EqPosBaseAlignAxisB=+Z  EqPosRotationSequenceAxes=FollowerAxes  EqPosRotationSequence=XYX  EqPosRotationSequenceAngles=[0 0 0]  EqPosRotationSequenceAnglesUnits=deg  EqPosRotationMatrix=[1 0 0; 0 1 0; 0 0 1]  EqPosQuaternion=[1 0 0 0]  SpringStiffness=0  SpringStiffnessUnits=N*m/deg  DampingCoefficient=0  DampingCoefficientUnits=N*m/(deg/s)  ActuateTorqueX=off  ActuateTorqueY=off  ActuateTorqueZ=off  ActuateTorque=off  TorqueActuationMode=NoTorque  MotionActuationMode=ComputedMotion  ActuationFrame=BaseFrame  SensePosition=off  SenseVelocityX=off  SenseVelocityY=off  SenseVelocityZ=off  SenseVelocity=off  SenseAccelerationX=off  SenseAccelerationY=off  SenseAccelerationZ=off  SenseAcceleration=off  SenseTorqueX=off  SenseTorqueY=off  SenseTorqueZ=off  SenseTorqueForce=off  SenseLowerLimitTorqueMag=off  SenseUpperLimitTorqueMag=off  SensingFrame=BaseFrame  LowerLimitSpecify=off  LowerLimitBound=15  LowerLimitBoundUnits=deg  LowerLimitStiffness=1e4  LowerLimitStiffnessUnits=N*m/deg  LowerLimitDamping=10  LowerLimitDampingUnits=N*m/(deg/s)  LowerLimitTransitionRegionWidth=0.1  LowerLimitTransitionRegionWidthUnits=deg  UpperLimitSpecify=off  UpperLimitBound=45  UpperLimitBoundUnits=deg  UpperLimitStiffness=1e4  UpperLimitStiffnessUnits=N*m/deg  UpperLimitDamping=10  UpperLimitDampingUnits=N*m/(deg/s)  UpperLimitTransitionRegionWidth=0.1  UpperLimitTransitionRegionWidthUnits=deg  PositionTargetRotationMethod=None  PositionTargetRotationAngleUnits=deg  PositionTargetRotationStandardAxis=+Z  PositionTargetRotationAngle=0.0  PositionTargetRotationArbitraryAxis=[0 0 1]  PositionTargetFollAlignAxisA=+X  PositionTargetBaseAlignAxisA=+Y  PositionTargetFollAlignAxisB=+Y  PositionTargetBaseAlignAxisB=+Z  PositionTargetRotationSequenceAxes=FollowerAxes  PositionTargetRotationSequence=XYX  PositionTargetRotationSequenceAngles=[0 0 0]  PositionTargetRotationSequenceAnglesUnits=deg  PositionTargetRotationMatrix=[1 0 0; 0 1 0; 0 0 1]  PositionTargetQuaternion=[1 0 0 0]  PositionTargetSpecify=off  PositionTargetPriority=High  VelocityTargetValue=[0 0 0]  VelocityTargetValueUnits=deg/s  VelocityTargetSpecify=off  VelocityTargetPriority=High  VelocityTargetInFollowerFrame=on
  Universal Joint{1..6} (6 alike) : sm_lib/Joints/Universal Joint  JointMode=Normal  SenseConstraintForce=off  SenseConstraintForceX=off  SenseConstraintForceY=off  SenseConstraintForceZ=off  SenseConstraintTorque=off  SenseConstraintTorqueX=off  SenseConstraintTorqueY=off  SenseConstraintTorqueZ=off  SenseTotalForce=off  SenseTotalForceX=off  SenseTotalForceY=off  SenseTotalForceZ=off  SenseTotalTorque=off  SenseTotalTorqueX=off  SenseTotalTorqueY=off  SenseTotalTorqueZ=off  CompositeWrenchDir=FollowerOnBase  CompositeWrenchFrame=BaseFrame  RxEquilibriumPosition=0  RxEquilibriumPositionUnits=deg  RxSpringStiffness=0  RxSpringStiffnessUnits=N*m/deg  RxDampingCoefficient=0  RxDampingCoefficientUnits=N*m/(deg/s)  RxTorqueActuationMode=NoTorque  RxMotionActuationMode=ComputedMotion  RxSensePosition=off  RxSenseVelocity=off  RxSenseAcceleration=off  RxSenseTorqueForce=off  RxSenseLowerLimitTorqueForce=off  RxSenseUpperLimitTorqueForce=off  RxLowerLimitSpecify=off  RxLowerLimitBound=-90  RxLowerLimitBoundUnits=deg  RxLowerLimitStiffness=1e4  RxLowerLimitStiffnessUnits=N*m/deg  RxLowerLimitDamping=10  RxLowerLimitDampingUnits=N*m/(deg/s)  RxLowerLimitTransitionRegionWidth=0.1  RxLowerLimitTransitionRegionWidthUnits=deg  RxUpperLimitSpecify=off  RxUpperLimitBound=90  RxUpperLimitBoundUnits=deg  RxUpperLimitStiffness=1e4  RxUpperLimitStiffnessUnits=N*m/deg  RxUpperLimitDamping=10  RxUpperLimitDampingUnits=N*m/(deg/s)  RxUpperLimitTransitionRegionWidth=0.1  RxUpperLimitTransitionRegionWidthUnits=deg  RxPositionTargetSpecify=off  RxPositionTargetPriority=High  RxPositionTargetValue=0  RxPositionTargetValueUnits=deg  RxVelocityTargetSpecify=off  RxVelocityTargetPriority=High  RxVelocityTargetValue=0  RxVelocityTargetValueUnits=deg/s  RyEquilibriumPosition=0  RyEquilibriumPositionUnits=deg  RySpringStiffness=0  RySpringStiffnessUnits=N*m/deg  RyDampingCoefficient=0  RyDampingCoefficientUnits=N*m/(deg/s)  RyTorqueActuationMode=NoTorque  RyMotionActuationMode=ComputedMotion  RySensePosition=off  RySenseVelocity=off  RySenseAcceleration=off  RySenseTorqueForce=off  RySenseLowerLimitTorqueForce=off  RySenseUpperLimitTorqueForce=off  RyLowerLimitSpecify=off  RyLowerLimitBound=-90  RyLowerLimitBoundUnits=deg  RyLowerLimitStiffness=1e4  RyLowerLimitStiffnessUnits=N*m/deg  RyLowerLimitDamping=10  RyLowerLimitDampingUnits=N*m/(deg/s)  RyLowerLimitTransitionRegionWidth=0.1  RyLowerLimitTransitionRegionWidthUnits=deg  RyUpperLimitSpecify=off  RyUpperLimitBound=90  RyUpperLimitBoundUnits=deg  RyUpperLimitStiffness=1e4  RyUpperLimitStiffnessUnits=N*m/deg  RyUpperLimitDamping=10  RyUpperLimitDampingUnits=N*m/(deg/s)  RyUpperLimitTransitionRegionWidth=0.1  RyUpperLimitTransitionRegionWidthUnits=deg  RyPositionTargetSpecify=off  RyPositionTargetPriority=High  RyPositionTargetValue=0  RyPositionTargetValueUnits=deg  RyVelocityTargetSpecify=off  RyVelocityTargetPriority=High  RyVelocityTargetValue=0  RyVelocityTargetValueUnits=deg/s
  Weld Joint{,1..5} (6 alike) : sm_lib/Joints/Weld Joint  JointMode=Normal  SenseConstraintForce=off  SenseConstraintForceX=off  SenseConstraintForceY=off  SenseConstraintForceZ=off  SenseConstraintTorque=off  SenseConstraintTorqueX=off  SenseConstraintTorqueY=off  SenseConstraintTorqueZ=off  SenseTotalForce=off  SenseTotalForceX=off  SenseTotalForceY=off  SenseTotalForceZ=off  SenseTotalTorque=off  SenseTotalTorqueX=off  SenseTotalTorqueY=off  SenseTotalTorqueZ=off  CompositeWrenchDir=FollowerOnBase  CompositeWrenchFrame=BaseFrame
  World Frame1 : sm_lib/Frames and Transforms/World Frame
  Conn1 : PMIOPort  Side=Left
  Conn2 : PMIOPort  Port=2  Side=Left
  Conn3 : PMIOPort  Port=3  Side=Left
  Conn4 : PMIOPort  Port=4  Side=Left
  Conn5 : PMIOPort  Port=5  Side=Left
  Conn6 : PMIOPort  Port=6  Side=Left
  connections:
  Prismatic Joint1/LConn1 -- Rigid Transform9/RConn1
  Revolved Solid4/LConn1 -- Universal Joint5/LConn1
  Weld Joint5/LConn1 -- Rigid Transform7/RConn1
  Prismatic Joint5/RConn1 -- Revolved Solid4/RConn1
  Rigid Transform20/LConn1 -- 6-DOF Joint/RConn1 -- Rigid Transform16/LConn1 -- Rigid Transform15/LConn1 -- Rigid Transform17/LConn1 -- Extruded Solid/RConn1 -- Rigid Transform18/LConn1 -- Rigid Transform19/LConn1
  Cylindrical Solid/RConn1 -- Rigid Transform8/LConn1
  Cylindrical Solid1/RConn1 -- Rigid Transform9/LConn1
  Cylindrical Solid7/RConn1 -- Spherical Joint2/LConn1
  Weld Joint4/LConn1 -- Rigid Transform6/RConn1
  Rigid Transform17/RConn1 -- Spherical Joint2/RConn1
  Revolved Solid3/LConn1 -- Universal Joint4/LConn1
  Cylindrical Solid/LConn1 -- Weld Joint/RConn1
  Prismatic Joint7/LConn2 -- Conn6/RConn1
  Cylindrical Solid5/RConn1 -- Rigid Transform13/LConn1
  Prismatic Joint3/RConn1 -- Revolved Solid2/RConn1
  Spherical Joint6/LConn1 -- Rigid Transform15/RConn1
  Cylindrical Solid12/LConn1 -- Universal Joint1/RConn1
  Cylindrical Solid9/LConn1 -- Universal Joint5/RConn1
  Prismatic Joint6/LConn2 -- Conn1/RConn1
  Prismatic Joint6/RConn1 -- Revolved Solid6/RConn1
  Cylindrical Solid4/RConn1 -- Rigid Transform12/LConn1
  Revolved Solid2/LConn1 -- Universal Joint3/LConn1
  Rigid Transform2/LConn1 -- World Frame1/RConn1 -- Mech Config1/RConn1 -- Rigid Transform14/LConn1 -- Extruded Solid2/RConn1 -- Solver Configuration/RConn1
  Cylindrical Solid10/LConn1 -- Universal Joint6/RConn1
  Cylindrical Solid4/LConn1 -- Weld Joint4/RConn1
  Cylindrical Solid12/RConn1 -- Spherical Joint6/RConn1
  Rigid Transform5/RConn1 -- Weld Joint3/LConn1
  Cylindrical Solid1/LConn1 -- Weld Joint1/RConn1
  Cylindrical Solid5/LConn1 -- Weld Joint5/RConn1
  Spherical Joint3/LConn1 -- Cylindrical Solid8/RConn1
  Universal Joint2/LConn1 -- Revolved Solid1/LConn1
  Cylindrical Solid6/RConn1 -- Spherical Joint1/RConn1
  Rigid Transform4/RConn1 -- Weld Joint2/LConn1
  Cylindrical Solid8/LConn1 -- Universal Joint4/RConn1
  Cylindrical Solid3/LConn1 -- Weld Joint3/RConn1
  Prismatic Joint1/RConn1 -- Revolved Solid1/RConn1
  Rigid Transform19/RConn1 -- Spherical Joint4/RConn1
  Prismatic Joint3/LConn2 -- Conn3/RConn1
  Weld Joint/LConn1 -- Rigid Transform3/RConn1
  Cylindrical Solid2/RConn1 -- Rigid Transform10/LConn1
  Prismatic Joint1/LConn2 -- Conn2/RConn1
  Prismatic Joint5/LConn1 -- Rigid Transform12/RConn1
  Cylindrical Solid9/RConn1 -- Spherical Joint4/LConn1
  Cylindrical Solid10/RConn1 -- Spherical Joint5/LConn1
  6-DOF Joint/LConn1 -- Rigid Transform14/RConn1
  Prismatic Joint3/LConn1 -- Rigid Transform10/RConn1
  Rigid Transform1/RConn1 -- Weld Joint1/LConn1
  Rigid Transform16/RConn1 -- Spherical Joint1/LConn1
  Prismatic Joint7/RConn1 -- Revolved Solid5/RConn1
  Cylindrical Solid6/LConn1 -- Universal Joint2/RConn1
  Rigid Transform18/RConn1 -- Spherical Joint3/RConn1
  Revolved Solid6/LConn1 -- Universal Joint1/LConn1
  Cylindrical Solid7/LConn1 -- Universal Joint3/RConn1
  Cylindrical Solid2/LConn1 -- Weld Joint2/RConn1
  Prismatic Joint4/LConn2 -- Conn4/RConn1
  Cylindrical Solid3/RConn1 -- Rigid Transform11/LConn1
  Revolved Solid5/LConn1 -- Universal Joint6/LConn1
  Rigid Transform20/RConn1 -- Spherical Joint5/RConn1
  Prismatic Joint7/LConn1 -- Rigid Transform13/RConn1
  Prismatic Joint4/RConn1 -- Revolved Solid3/RConn1
  Prismatic Joint6/LConn1 -- Rigid Transform8/RConn1
  Prismatic Joint4/LConn1 -- Rigid Transform11/RConn1
  Rigid Transform4/LConn1 -- Rigid Transform3/LConn1 -- Rigid Transform2/RConn1 -- Rigid Transform1/LConn1 -- Rigid Transform7/LConn1 -- Rigid Transform6/LConn1 -- Rigid Transform5/LConn1
  Prismatic Joint5/LConn2 -- Conn5/RConn1

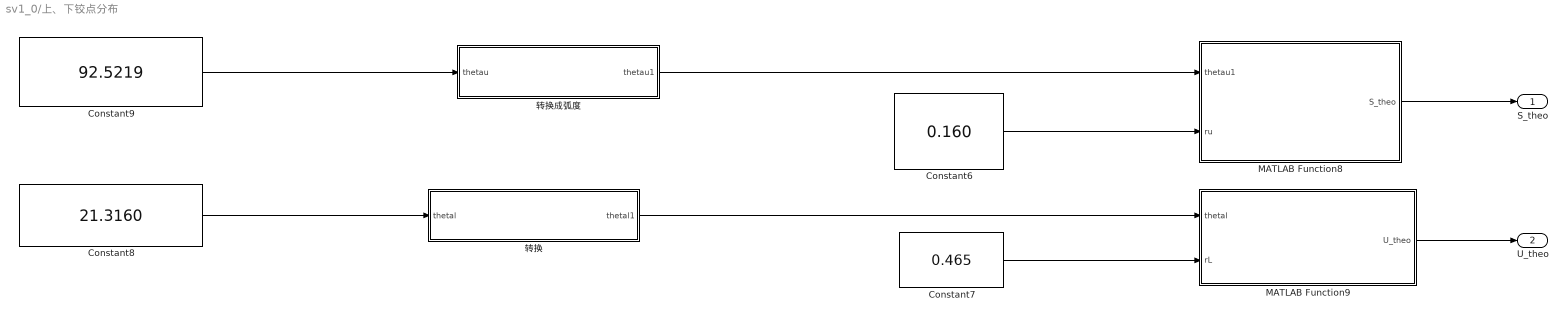
== system sv1_0/上、下铰点分布 ==
  Constant6 : Constant  Value=0.160
  Constant7 : Constant  Value=0.465
  Constant8 : Constant  Value=21.3160
  Constant9 : Constant  Value=92.5219
  MATLAB Function8 : MATLAB Function  TreatAsAtomicUnit=on
  MATLAB Function9 : MATLAB Function  TreatAsAtomicUnit=on
  转换 : MATLAB Function  TreatAsAtomicUnit=on
  转换成弧度 : MATLAB Function  TreatAsAtomicUnit=on
  S_theo : Outport
  U_theo : Outport  Port=2
  wires:
  Constant9/1 -> 转换成弧度/1(thetau)
  转换成弧度/1(thetau1) -> MATLAB Function8/1(thetau1)
  Constant6/1 -> MATLAB Function8/2(ru)
  转换/1(thetal1) -> MATLAB Function9/1(thetal)
  MATLAB Function9/1(U_theo) -> U_theo/1
  Constant7/1 -> MATLAB Function9/2(rL)
  MATLAB Function8/1(S_theo) -> S_theo/1
  Constant8/1 -> 转换/1(thetal)

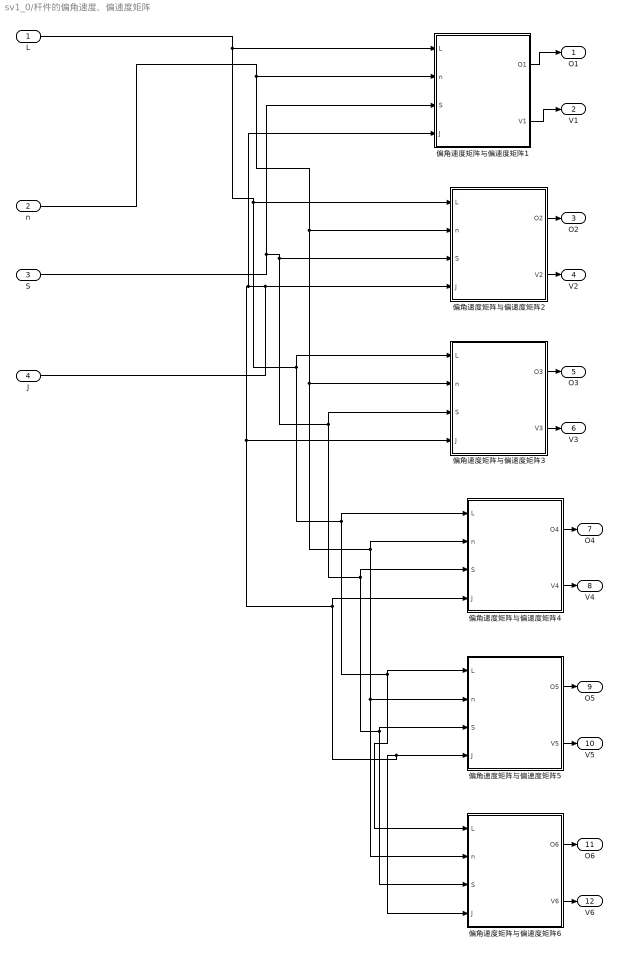
== system sv1_0/杆件的偏角速度、偏速度矩阵 ==
  L : Inport
  n : Inport  Port=2
  S : Inport  Port=3
  J : Inport  Port=4
  偏角速度矩阵与偏速度矩阵1 : MATLAB Function  TreatAsAtomicUnit=on
  偏角速度矩阵与偏速度矩阵2 : MATLAB Function  TreatAsAtomicUnit=on
  偏角速度矩阵与偏速度矩阵3 : MATLAB Function  TreatAsAtomicUnit=on
  偏角速度矩阵与偏速度矩阵4 : MATLAB Function  TreatAsAtomicUnit=on
  偏角速度矩阵与偏速度矩阵5 : MATLAB Function  TreatAsAtomicUnit=on
  偏角速度矩阵与偏速度矩阵6 : MATLAB Function  TreatAsAtomicUnit=on
  O1 : Outport
  V1 : Outport  Port=2
  O2 : Outport  Port=3
  V2 : Outport  Port=4
  O3 : Outport  Port=5
  V3 : Outport  Port=6
  O4 : Outport  Port=7
  V4 : Outport  Port=8
  O5 : Outport  Port=9
  V5 : Outport  Port=10
  O6 : Outport  Port=11
  V6 : Outport  Port=12
  wires:
  偏角速度矩阵与偏速度矩阵6/1(O6) -> O6/1
  S/1 -> 偏角速度矩阵与偏速度矩阵1/3(S), 偏角速度矩阵与偏速度矩阵6/3(S), 偏角速度矩阵与偏速度矩阵5/3(S), 偏角速度矩阵与偏速度矩阵4/3(S), 偏角速度矩阵与偏速度矩阵3/3(S), 偏角速度矩阵与偏速度矩阵2/3(S)
  J/1 -> 偏角速度矩阵与偏速度矩阵1/4(J), 偏角速度矩阵与偏速度矩阵4/4(J), 偏角速度矩阵与偏速度矩阵5/4(J), 偏角速度矩阵与偏速度矩阵6/4(J), 偏角速度矩阵与偏速度矩阵3/4(J), 偏角速度矩阵与偏速度矩阵2/4(J)
  n/1 -> 偏角速度矩阵与偏速度矩阵1/2(n), 偏角速度矩阵与偏速度矩阵2/2(n), 偏角速度矩阵与偏速度矩阵4/2(n), 偏角速度矩阵与偏速度矩阵6/2(n), 偏角速度矩阵与偏速度矩阵5/2(n), 偏角速度矩阵与偏速度矩阵3/2(n)
  偏角速度矩阵与偏速度矩阵1/1(O1) -> O1/1
  L/1 -> 偏角速度矩阵与偏速度矩阵6/1(L), 偏角速度矩阵与偏速度矩阵5/1(L), 偏角速度矩阵与偏速度矩阵4/1(L), 偏角速度矩阵与偏速度矩阵3/1(L), 偏角速度矩阵与偏速度矩阵2/1(L), 偏角速度矩阵与偏速度矩阵1/1(L)
  偏角速度矩阵与偏速度矩阵2/1(O2) -> O2/1
  偏角速度矩阵与偏速度矩阵2/2(V2) -> V2/1
  偏角速度矩阵与偏速度矩阵1/2(V1) -> V1/1
  偏角速度矩阵与偏速度矩阵4/1(O4) -> O4/1
  偏角速度矩阵与偏速度矩阵5/1(O5) -> O5/1
  偏角速度矩阵与偏速度矩阵5/2(V5) -> V5/1
  偏角速度矩阵与偏速度矩阵6/2(V6) -> V6/1
  偏角速度矩阵与偏速度矩阵3/1(O3) -> O3/1
  偏角速度矩阵与偏速度矩阵4/2(V4) -> V4/1
  偏角速度矩阵与偏速度矩阵3/2(V3) -> V3/1

== matlab function sv1_0/上、下铰点分布/MATLAB Function8 ==
  data: S_theo output; thetau1 input; ru input
function S_theo= fcn(thetau1,ru)
S_theo=zeros(3,6);
for i= 1 : 1 : 3 
S_theo(1,2*i-1)= ru * cos(pi*2/3*(i-1) + pi/2 - thetau1/2);
S_theo(2,2*i-1)= ru * sin(pi*2/3*(i-1) + pi/2 - thetau1/2);
S_theo(3,2*i-1)= 0;
S_theo(1,2*i)= ru * cos(pi*2/3*(i-1) + pi/2 + thetau1/2);
S_theo(2,2*i)= ru * sin(pi*2/3*(i-1) + pi/2 + thetau1/2);
S_theo(3,2*i)= 0;
end

== matlab function sv1_0/上、下铰点分布/MATLAB Function9 ==
  data: U_theo output; thetal input; rL input
function U_theo= fcn(thetal,rL)
U_theo=zeros(3,6);
for i= 1 : 1 : 3 
U_theo(1,2*i-1)= rL * cos(pi*2/3*(i-1) + pi/2 - thetal/2);
U_theo(2,2*i-1)= rL * sin(pi*2/3*(i-1) + pi/2 - thetal/2);
U_theo(3,2*i-1)= 0;
U_theo(1,2*i)= rL * cos(pi*2/3*(i-1) + pi/2 + thetal/2);
U_theo(2,2*i)= rL * sin(pi*2/3*(i-1) + pi/2 + thetal/2);
U_theo(3,2*i)= 0;
end

== matlab function sv1_0/上、下铰点分布/转换成弧度 ==
  data: thetau1 output; thetau input
function thetau1= fcn(thetau)
thetau1=(thetau/180)*pi;

== matlab function sv1_0/上、下铰点分布/转换 ==
  data: thetal1 output; thetal input
function thetal1= fcn(thetal)
thetal1=(thetal/180)*pi;

== matlab function sv1_0/杆件的偏角速度、偏速度矩阵/偏角速度矩阵与偏速度矩阵4 ==
  data: L input; n input; S input; J input; O4 output; V4 output
function [O4,V4]=fcn(L,n,S,J)
OO1=zeros(1,6);
E=eye(3,3);
s=skew(S(:,4));%求反对称矩阵
OO3=J(4,:);
OO4=[OO1;OO1;OO3];
O4=skew((n(:,4)/L))*([E,s]-OO4);%杆件偏角速度
V4=OO4-L/2*skew((n(:,4)))*O4;%杆件偏速度

== matlab function sv1_0/杆件的偏角速度、偏速度矩阵/偏角速度矩阵与偏速度矩阵5 ==
  data: L input; n input; S input; J input; O5 output; V5 output
function [O5,V5]=fcn(L,n,S,J)
OO1=zeros(1,6);
E=eye(3,3);
s=skew(S(:,5));%求反对称矩阵
OO3=J(5,:);
OO4=[OO1;OO1;OO3];
O5=skew((n(:,5)/L))*([E,s]-OO4);%杆件偏角速度
V5=OO4-L/2*skew((n(:,2)))*O5;%杆件偏速度

== matlab function sv1_0/杆件的偏角速度、偏速度矩阵/偏角速度矩阵与偏速度矩阵6 ==
  data: L input; n input; S input; J input; O6 output; V6 output
function [O6,V6]=fcn(L,n,S,J)
OO1=zeros(1,6);
E=eye(3,3);
s=skew(S(:,6));%求反对称矩阵
OO3=J(6,:);
OO4=[OO1;OO1;OO3];
O6=skew((n(:,6)/L))*([E,s]-OO4);%杆件偏角速度
V6=OO4-L/2*skew((n(:,6)))*O6;%杆件偏速度

== matlab function sv1_0/角速度 ==
  data: n input; S input; J output
function J =fcn(n,S)
e=[0,0,1];
J=zeros(6,6);
s=zeros(3,3)
for i=1:6
s=skew(S(:,i));%求反对称矩阵
K=e*n(:,i);
J(i,:)=[n(:,i)'/K,(s*n(:,i))'/K];
end

== matlab function sv1_0/位置反解与方向向量 ==
  data: L input; q output; p input; TR input; S_theo input; U_theo input; n output; S output
function [q,n,S]= fcn(L,p, TR,S_theo,U_theo)
d=zeros(3,6);
q=zeros(1,6);
n=zeros(3,6);
e=[0,0,1];
S=zeros(3,6);
for i=1:6
S(:,i)=TR*S_theo(:,i);%上铰点在惯性坐标下的坐标
d(:,i) =  S(:,i)+p-U_theo(:,i);
q(i)= e*d(:,i)-sqrt((e*d(:,i))^2-d(:,i)'*d(:,i)+L^2);
n(:,i)=(p+d(:,i) -q(i)*e')/L;
end

== matlab function sv1_0/旋转矩阵TR ==
  data: TR output; alpha_in input; beta_in input; gamma_in input
function TR = fcn(alpha_in,beta_in,gamma_in)
R=zeros(3,3);
R(1,1)=cos(beta_in)*cos(gamma_in);
R(1,2)=sin(beta_in)*cos(gamma_in)*sin(alpha_in)-cos(alpha_in)*sin(gamma_in);
R(1,3)=sin(alpha_in)*sin(gamma_in)+cos(gamma_in)*cos(alpha_in)*sin(beta_in);
R(2,1)=cos(alpha_in)*sin(gamma_in);
R(2,2)=-sin(alpha_in)*sin(beta_in)*sin(gamma_in)+cos(alpha_in)*cos(gamma_in);
R(2,3)=cos(alpha_in)*sin(beta_in)*sin(gamma_in)-sin(alpha_in)*cos(gamma_in);
R(3,1)=-sin(beta_in);
R(3,2)=sin(alpha_in)*cos(beta_in);
R(3,3)=cos(alpha_in)*cos(beta_in);
TR=R;

== matlab function sv1_0/平移向量P ==
  data: z0 input; p output; x_in input; y_in input; z_in input
function p= fcn(z0,x_in,y_in,z_in)

p=[x_in;y_in;z_in+z0];

== matlab function sv1_0/总体雅可比矩阵 ==
  data: n input; S input; J output
function J =fcn(n,S)
e=[0,0,1];
J=zeros(6,6);
s=zeros(3,3)
for i=1:6
s=skew(S(:,i));%求反对称矩阵
K=e*n(:,i);
J(i,:)=[n(:,i)'/K,(s*n(:,i))'/K];
end

== matlab function sv1_0/角速度与欧拉角变化率转换关系 ==
  data: B output; alpha_in input; beta_in input
function B= fcn(alpha_in,beta_in)
 B=[1,0,-sin(beta_in);
    0,cos(alpha_in),sin(alpha_in)*cos(beta_in);
    0,-sin(alpha_in),cos(alpha_in)*cos(beta_in)];

== matlab function sv1_0/杆件的偏角速度、偏速度矩阵/偏角速度矩阵与偏速度矩阵1 ==
  data: L input; n input; S input; J input; O1 output; V1 output
function [O1,V1]=fcn(L,n,S,J)
OO1=zeros(1,6);
E=eye(3,3);
s=skew(S(:,1));%求反对称矩阵
OO3=J(1,:);
OO4=[OO1;OO1;OO3];
O1=skew((n(:,1)/L))*([E,s]-OO4);%杆件偏角速度
V1=OO4-L/2*skew((n(:,1)))*O1;%杆件偏速度
